simulink model "sampleModel1908"  (R2023a)
settings: Solver=VariableStepAuto  StartTime=0.0  StopTime=10.0  RelTol=1e-3
libraries: hdlsllib x9, simulink x3
settings Model: Creator=user1  LastModifiedBy=user1

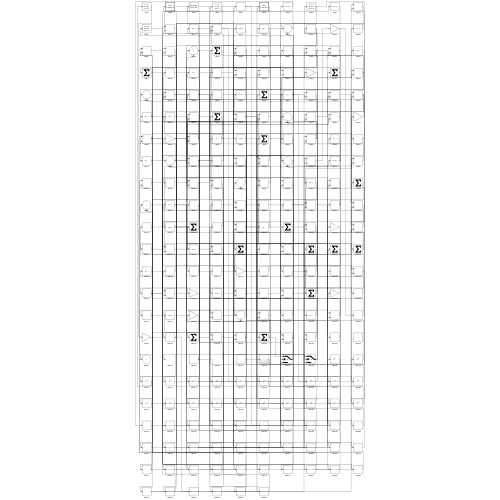
[thumbnail: Simulink's stored preview of the top-level diagram]
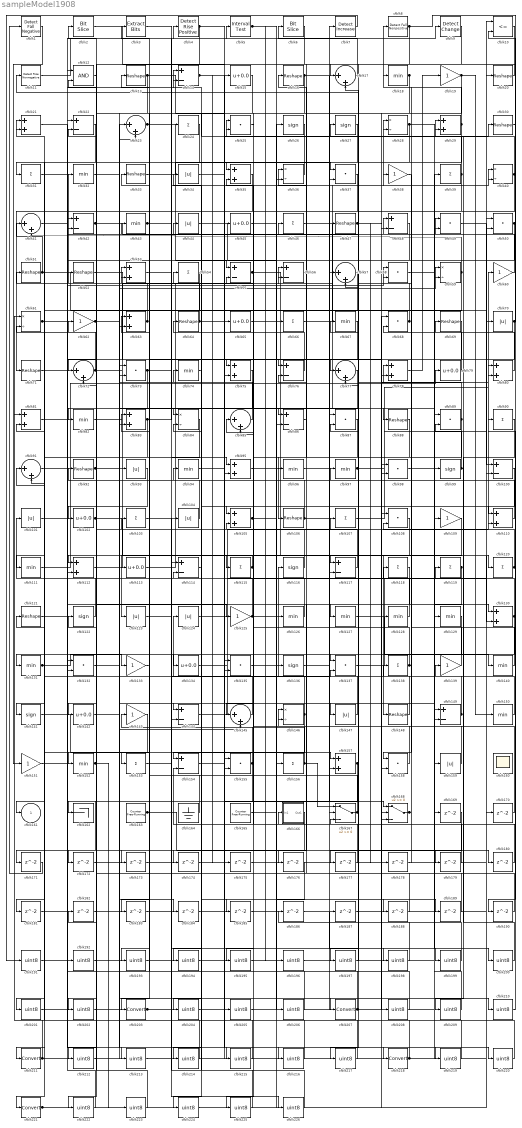
== system sampleModel1908 ==
  cfblk1 : hdlsllib/Logic and Bit Operations/Detect Fall Negative  vinit=0  OutDataTypeStr=boolean
  cfblk10 : RelationalOperator  Operator=<=  OutDataTypeStr=boolean  InputSameDT=off
  cfblk{14,22,42,48,55..56,76,86,100,114,117,144,149,154} (14 alike) : Sum  Inputs=+-
  cfblk{34,44,70,93,101,104,123..124,147,159} (10 alike) : Abs  SaturateOnIntegerOverflow=off
  cfblk{15,45,65,79,102,113,134,142} (8 alike) : Bias  Bias=0.0  SaturateOnIntegerOverflow=off
  cfblk{24,31,39,46,54,66,90,103,107,115,118..120,138,153,156} (16 alike) : Sum  Inputs=+
  cfblk{21,29,35,53,63,75,78,80..81,83,95,105,110,112,130,157} (16 alike) : Sum
  cfblk{13,16,20,30,33,47,51..52,64,69,71,88,92,106,121,148} (16 alike) : Reshape
  cfblk{25,37,49..50,58,68,73,87,89,98,108,132,135,137,155,158} (16 alike) : DotProduct  OutDataTypeStr=Inherit: Inherit via internal rule
  cfblk{19,38,60,62,109,125,133,139,143,151} (10 alike) : Gain
  cfblk11 : hdlsllib/Logic and Bit Operations/Detect Rise Nonnegative  vinit=0  OutDataTypeStr=boolean
  cfblk{18,32,43,67,74,82,94,96..97,111,126..129,131,140,150,152} (18 alike) : MinMax
  cfblk{26..27,99,116,122,136,141} (7 alike) : Signum
  cfblk12 : Logic  AllPortsSameDT=off  OutDataTypeStr=boolean
  cfblk{17,23,41,57,72,77,85,91,145} (9 alike) : Sum  Inputs=|++
  cfblk{28,36,40,59,61,84,146} (7 alike) : Product  Inputs=*/  RndMeth=Zero  SaturateOnIntegerOverflow=on
  cfblk160 : Scope
      settings: Floating=on
  cfblk162 : Terminator
  cfblk163 : hdlsllib/Sources/Counter Free-Running  NumBits=16  tsamp=-1
  cfblk164 : Ground
  cfblk165 : hdlsllib/Sources/Counter Free-Running  NumBits=16  tsamp=-1
  cfblk166 : Subsystem
      settings: LibrarySourceBlock=|
      | hdlsllib/Ports &
      | Subsystems/Subsystem
  cfblk167 : Switch  SaturateOnIntegerOverflow=off  InputSameDT=off
  cfblk168 : Switch  SaturateOnIntegerOverflow=off  InputSameDT=off
  cfblk{169..190} (22 alike) : Delay  SampleTime=1
  cfblk{191..202,204..206,208..210,212..217,219..220,222..226} (31 alike) : DataTypeConversion  OutDataTypeStr=uint8  SaturateOnIntegerOverflow=off  RndMeth=Floor
  cfblk2 : hdlsllib/Logic and Bit Operations/Bit Slice  lidx=7  ridx=0
  cfblk{203,207,211,218,221} (5 alike) : DataTypeConversion  SaturateOnIntegerOverflow=off  RndMeth=Floor
  cfblk3 : simulink/Logic and Bit Operations/Extract Bits  bitsToExtract=Upper half  numBits=8  bitIdxRange=[0 7]  outScalingMode=Preserve fixed-point scaling
      settings: LibrarySourceBlock=|
      | hdlsllib/Logic and Bit
      | Operations/Extract Bits
  cfblk4 : hdlsllib/Logic and Bit Operations/Detect Rise Positive  vinit=0  OutDataTypeStr=boolean
  cfblk5 : hdlsllib/Logic and Bit Operations/Interval Test  IntervalClosedRight=on  uplimit=0.5  IntervalClosedLeft=on  lowlimit=-0.5  OutDataTypeStr=boolean
  cfblk6 : hdlsllib/Logic and Bit Operations/Bit Slice  lidx=7  ridx=0
  cfblk7 : simulink/Logic and Bit Operations/Detect Increase  vinit=0.0  OutDataTypeStr=boolean
      settings: LibrarySourceBlock=|
      | hdlsllib/Logic and Bit
      | Operations/Detect
      | Increase
  cfblk8 : hdlsllib/Logic and Bit Operations/Detect Fall Nonpositive  vinit=0  OutDataTypeStr=boolean
  cfblk9 : simulink/Logic and Bit Operations/Detect Change  vinit=0  OutDataTypeStr=boolean
      settings: LibrarySourceBlock=|
      | hdlsllib/Logic and Bit
      | Operations/Detect
      | Change
  cfblk161 : Outport  VectorParamsAs1DForOutWhenUnconnected=off
  wires:
  cfblk37/1 -> cfblk71/1
  cfblk64/1 -> cfblk32/1, cfblk30/1
  cfblk42/1 -> cfblk27/1, cfblk144/1
  cfblk147/1 -> cfblk116/1
  cfblk111/1 -> cfblk79/1
  cfblk113/1 -> cfblk56/1
  cfblk61/1 -> cfblk58/1, cfblk219/1
  cfblk131/1 -> cfblk133/1, cfblk14/1
  cfblk23/1 -> cfblk55/1, cfblk113/1
  cfblk97/1 -> cfblk60/1, cfblk80/2
  cfblk36/1 -> cfblk35/1
  cfblk10/1 -> cfblk36/1
  cfblk124/1 -> cfblk107/1
  cfblk138/1 -> cfblk35/2, cfblk108/2
  cfblk48/1 -> cfblk105/1
  cfblk78/1 -> cfblk19/1
  cfblk95/1 -> cfblk148/1
  cfblk130/1 -> cfblk137/1, cfblk77/2
  cfblk40/1 -> cfblk29/1, cfblk57/2, cfblk14/2, cfblk201/1
  cfblk18/1 -> cfblk48/2, cfblk204/1
  cfblk141/1 -> cfblk157/1
  cfblk67/1 -> cfblk115/1
  cfblk68/1 -> cfblk25/1, cfblk11/1
  cfblk55/1 -> cfblk149/1, cfblk149/2
  cfblk56/1 -> cfblk16/1
  cfblk33/1 -> cfblk37/1
  cfblk163/1 -> cfblk33/1, cfblk208/1
  cfblk63/1 -> cfblk53/1, cfblk53/2
  cfblk72/1 -> cfblk54/1, cfblk59/2, cfblk61/2
  cfblk102/1 -> cfblk28/1, cfblk128/1, cfblk130/2
  cfblk5/1 -> cfblk168/3, cfblk196/1
  cfblk165/1 -> cfblk66/1
  cfblk16/1 -> cfblk102/1, cfblk168/2
  cfblk108/1 -> cfblk123/1
  cfblk112/1 -> cfblk56/2
  cfblk137/1 -> cfblk119/1
  cfblk89/1 -> cfblk127/1, cfblk17/2
  cfblk31/1 -> cfblk75/1
  cfblk50/1 -> cfblk84/1, cfblk112/2, cfblk190/1
  cfblk44/1 -> cfblk156/1
  cfblk39/1 -> cfblk25/2, cfblk135/2
  cfblk167/1 -> cfblk146/1, cfblk83/1
  cfblk1/1 -> cfblk151/1
  cfblk29/1 -> cfblk8/1, cfblk144/2
  cfblk17/1 -> cfblk6/1
  cfblk14/1 -> cfblk37/2, cfblk175/1
  cfblk117/1 -> cfblk105/2
  cfblk164/1 -> cfblk13/1
  cfblk145/1 -> cfblk74/1
  cfblk28/1 -> cfblk131/1, cfblk130/1, cfblk96/1
  cfblk27/1 -> cfblk153/1
  cfblk106/1 -> cfblk92/1, cfblk40/2
  cfblk22/1 -> cfblk221/1
  cfblk11/1 -> cfblk4/1
  cfblk82/1 -> cfblk24/1
  cfblk84/1 -> cfblk141/1
  cfblk83/1 -> cfblk9/1, cfblk161/1
  cfblk2/1 -> cfblk65/1
  cfblk53/1 -> cfblk95/1
  cfblk15/1 -> cfblk203/1
  cfblk125/1 -> cfblk36/2, cfblk21/2
  cfblk156/1 -> cfblk143/1, cfblk167/1
  cfblk86/1 -> cfblk46/1
  cfblk47/1 -> cfblk178/1, cfblk179/1
  cfblk59/1 -> cfblk117/1, cfblk41/2
  cfblk134/1 -> cfblk118/1
  cfblk79/1 -> cfblk76/1, cfblk48/1
  cfblk62/1 -> cfblk23/2, cfblk147/1, cfblk202/1
  cfblk88/1 -> cfblk106/1
  cfblk120/1 -> cfblk80/1, cfblk58/2
  cfblk92/1 -> cfblk145/2, cfblk210/1
  cfblk13/1 -> cfblk45/1, cfblk83/2
  cfblk150/1 -> cfblk29/2
  cfblk105/1 -> cfblk188/1, cfblk189/1
  cfblk158/1 -> cfblk51/1
  cfblk152/1 -> cfblk12/2, cfblk223/1
  cfblk85/1 -> cfblk3/1
  cfblk146/1 -> cfblk154/1, cfblk122/1
  cfblk99/1 -> cfblk49/1, cfblk89/2
  cfblk122/1 -> cfblk101/1
  cfblk21/1 -> cfblk132/1
  cfblk140/1 -> cfblk68/2
  cfblk35/1 -> cfblk95/2
  cfblk32/1 -> cfblk88/1
  cfblk6/1 -> cfblk82/1
  cfblk74/1 -> cfblk34/1
  cfblk46/1 -> cfblk159/1
  cfblk45/1 -> cfblk136/1
  cfblk8/1 -> cfblk166/1(In1), cfblk217/1
  cfblk128/1 -> cfblk43/1
  cfblk110/1 -> cfblk42/1
  cfblk66/1 -> cfblk38/1
  cfblk9/1 -> cfblk152/1
  cfblk126/1 -> cfblk62/1
  cfblk139/1 -> cfblk78/1
  cfblk52/1 -> cfblk77/1
  cfblk107/1 -> cfblk50/2
  cfblk153/1 -> cfblk137/2
  cfblk51/1 -> cfblk100/1, cfblk41/1
  cfblk127/1 -> cfblk140/1
  cfblk26/1 -> cfblk73/2
  cfblk119/1 -> cfblk176/1, cfblk177/1
  cfblk168/1 -> cfblk138/1, cfblk18/1
  cfblk70/1 -> cfblk10/2, cfblk185/1
  cfblk73/1 -> cfblk142/1, cfblk40/1, cfblk59/1
  cfblk155/1 -> cfblk64/1, cfblk194/1
  cfblk24/1 -> cfblk31/1
  cfblk159/1 -> cfblk97/1
  cfblk80/1 -> cfblk69/1
  cfblk118/1 -> cfblk162/1
  cfblk149/1 -> cfblk124/1, cfblk85/1
  cfblk96/1 -> cfblk47/1
  cfblk157/1 -> cfblk67/1, cfblk172/1
  cfblk71/1 -> cfblk52/1
  cfblk103/1 -> cfblk207/1
  cfblk116/1 -> cfblk42/2
  cfblk30/1 -> cfblk110/1
  cfblk136/1 -> cfblk110/2
  cfblk129/1 -> cfblk211/1
  cfblk91/1 -> cfblk218/1
  cfblk100/1 -> cfblk134/1
  cfblk148/1 -> cfblk21/1
  cfblk20/1 -> cfblk17/1
  cfblk151/1 -> cfblk5/1
  cfblk38/1 -> cfblk158/1
  cfblk115/1 -> cfblk112/1, cfblk85/2
  cfblk54/1 -> cfblk111/1
  cfblk93/1 -> cfblk132/2
  cfblk60/1 -> cfblk2/1
  cfblk76/1 -> cfblk44/1
  cfblk4/1 -> cfblk72/1, cfblk168/1
  cfblk144/1 -> cfblk100/2
  cfblk43/1 -> cfblk78/2, cfblk86/1
  cfblk41/1 -> cfblk125/1
  cfblk65/1 -> cfblk120/1
  cfblk19/1 -> cfblk145/1, cfblk150/1
  cfblk104/1 -> cfblk63/1
  cfblk57/1 -> cfblk63/2
  cfblk49/1 -> cfblk70/1
  cfblk58/1 -> cfblk39/1
  cfblk170/1 -> cfblk73/1
  cfblk143/1 -> cfblk171/1
  cfblk171/1 -> cfblk1/1
  cfblk172/1 -> cfblk75/2
  cfblk133/1 -> cfblk173/1
  cfblk173/1 -> cfblk50/1
  cfblk77/1 -> cfblk174/1
  cfblk174/1 -> cfblk84/2
  cfblk175/1 -> cfblk167/2
  cfblk177/1 -> cfblk154/2
  cfblk178/1 -> cfblk28/2
  cfblk179/1 -> cfblk76/2
  cfblk34/1 -> cfblk180/1
  cfblk180/1 -> cfblk55/2
  cfblk166/1(Out1) -> cfblk181/1
  cfblk181/1 -> cfblk23/1
  cfblk182/1 -> cfblk155/1
  cfblk69/1 -> cfblk183/1
  cfblk183/1 -> cfblk157/2
  cfblk132/1 -> cfblk184/1
  cfblk184/1 -> cfblk10/1
  cfblk185/1 -> cfblk86/2
  cfblk187/1 -> cfblk68/1
  cfblk188/1 -> cfblk146/2
  cfblk189/1 -> cfblk167/3
  cfblk190/1 -> cfblk72/2
  cfblk7/1 -> cfblk191/1
  cfblk191/1 -> cfblk104/1
  cfblk101/1 -> cfblk192/1
  cfblk192/1 -> cfblk7/1
  cfblk109/1 -> cfblk193/1
  cfblk193/1 -> cfblk169/1
  cfblk194/1 -> cfblk109/1
  cfblk87/1 -> cfblk195/1
  cfblk195/1 -> cfblk26/1
  cfblk196/1 -> cfblk87/1
  cfblk169/1 -> cfblk197/1
  cfblk197/1 -> cfblk87/2
  cfblk186/1 -> cfblk198/1
  cfblk198/1 -> cfblk108/1
  cfblk123/1 -> cfblk199/1
  cfblk199/1 -> cfblk186/1
  cfblk98/1 -> cfblk200/1
  cfblk200/1 -> cfblk139/1
  cfblk201/1 -> cfblk98/1
  cfblk202/1 -> cfblk98/2
  cfblk203/1 -> cfblk187/1, cfblk117/2, cfblk57/1
  cfblk204/1 -> cfblk15/1
  cfblk94/1 -> cfblk205/1
  cfblk205/1 -> cfblk49/2
  cfblk135/1 -> cfblk206/1
  cfblk206/1 -> cfblk94/1
  cfblk207/1 -> cfblk99/1, cfblk12/1
  cfblk208/1 -> cfblk103/1
  cfblk90/1 -> cfblk209/1
  cfblk209/1 -> cfblk89/1
  cfblk210/1 -> cfblk90/1
  cfblk211/1 -> cfblk61/1, cfblk93/1
  cfblk12/1 -> cfblk212/1
  cfblk212/1 -> cfblk129/1
  cfblk81/1 -> cfblk213/1
  cfblk213/1 -> cfblk155/2
  cfblk176/1 -> cfblk214/1
  cfblk214/1 -> cfblk81/1
  cfblk142/1 -> cfblk215/1
  cfblk215/1 -> cfblk81/2
  cfblk121/1 -> cfblk216/1
  cfblk216/1 -> cfblk182/1
  cfblk217/1 -> cfblk121/1
  cfblk218/1 -> cfblk135/1, cfblk20/1
  cfblk219/1 -> cfblk91/1
  cfblk154/1 -> cfblk220/1
  cfblk220/1 -> cfblk91/2
  cfblk221/1 -> cfblk158/2, cfblk126/1
  cfblk75/1 -> cfblk222/1
  cfblk222/1 -> cfblk22/1
  cfblk223/1 -> cfblk22/2
  cfblk114/1 -> cfblk224/1
  cfblk224/1 -> cfblk170/1
  cfblk25/1 -> cfblk225/1
  cfblk225/1 -> cfblk114/1
  cfblk3/1 -> cfblk226/1
  cfblk226/1 -> cfblk114/2

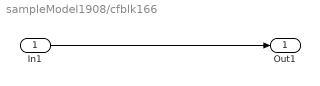
== system sampleModel1908/cfblk166 ==
  In1 : Inport
  Out1 : Outport
  wires:
  In1/1 -> Out1/1
